simulink model "control_volume_two_phases_test01_sim"  (R2017b)
settings: Solver=ode23tb  StartTime=0.0  StopTime=400  MaxStep=0.2  RelTol=1e-3
undefined symbols (not defined in the file or in its folder): h, P, T
libraries: thermochemical x6, simulink x2
settings Model: Creator=ferru  LastModifiedBy=fferrucc
settings SolverCC: AlgebraicLoopSolver=LineSearch

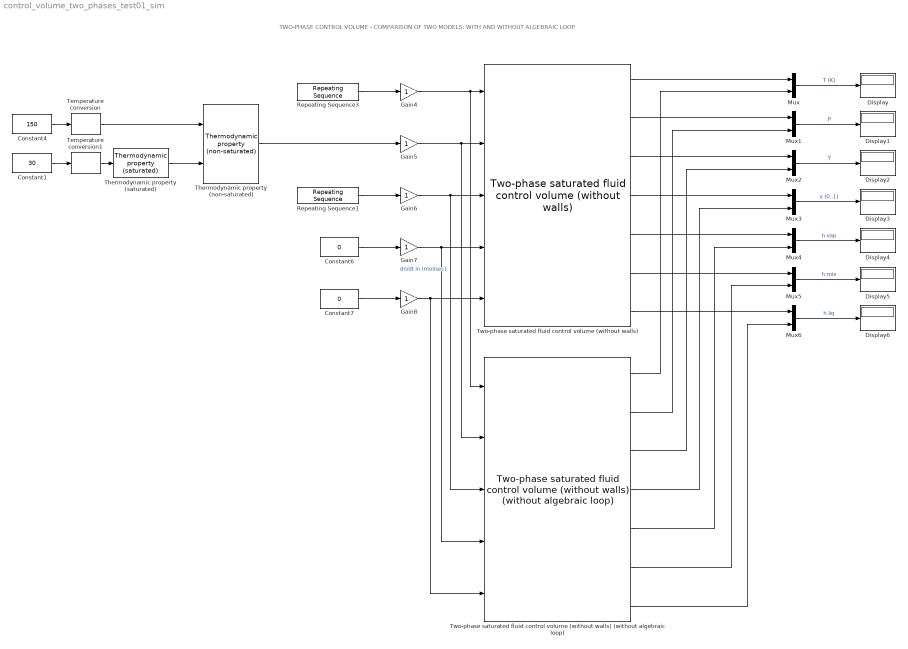
== system control_volume_two_phases_test01_sim ==
  note: TWO-PHASE CONTROL VOLUME - COMPARISON OF TWO MODELS: WITH AND WITHOUT ALGEBRAIC LOOP
  Constant1 : Constant  Value=30
  Constant4 : Constant  Value=150
  Constant6 : Constant  Value=0
  Constant7 : Constant  Value=0
  Display{,1..6} (7 alike) : Display
  Gain{4..8} (5 alike) : Gain
  Mux{,1..6} (7 alike) : Mux  Inputs=2
  Repeating Sequence1 : simulink/Sources/Repeating Sequence  rep_seq_t=[0, 100, 101, 200, 201]  rep_seq_y=[0, 0, 1, 1, 0]*0.02
  Repeating Sequence3 : simulink/Sources/Repeating Sequence  rep_seq_t=[0, 100, 101, 200, 201]  rep_seq_y=[1, 1, 0, 0, 1]*100
  Temperature conversion : thermochemical/Conversions/Temperature conversion  sel=°C --> K
      settings: SourceProductName=@ Thermochemical
  Temperature conversion1 : thermochemical/Conversions/Temperature conversion  sel=°C --> K
      settings: SourceProductName=@ Thermochemical
  Thermodynamic property (non-saturated) : thermochemical/Thermodynamic fluid properties/Thermodynamic  property (non-saturated)  sel=h(T,P)  fluid=nh3_v4  reciprocVar=-1  lookup2D_BreakPoint1=nh3_v4.no_sat.T_P_indep.var_indep.T  lookup2D_BreakPoint2=nh3_v4.no_sat.T_P_indep.var_indep.P  lookup2D_Data=nh3_v4.no_sat.T_P_indep.var_dep.h_molar
      settings: SourceProductName=@ Thermochemical
  Thermodynamic property (saturated) : thermochemical/Thermodynamic fluid properties/Thermodynamic  property (saturated)  sel=P(T) (bar)  fluid=nh3_v4  lookup1D_BreakPoint1=nh3_v4.sat.T  lookup1D_Data=nh3_v4.sat.Psat
      settings: SourceProductName=@ Thermochemical
  Two-phase saturated fluid control volume (without walls) : thermochemical/Control volumes/Two-phase saturated fluid control volume (without walls)  N_init=100  T_init=300  fluid=nh3_v4  V=0.01
      settings: SourceProductName=@ Thermochemical
  Two-phase saturated fluid control volume (without walls) (without algebraic loop) : thermochemical/Control volumes/Two-phase saturated fluid control volume (without walls) (without algebraic loop)  N_init=100  T_init=300  fluid=nh3_v4  V=0.01
      settings: SourceProductName=@ Thermochemical
  wires:
  Thermodynamic property (non-saturated)/1 -> Gain5/1
  Mux/1 -> Display/1  "T (K)"
  Two-phase saturated fluid control volume (without walls)/1 -> Mux/1
  Two-phase saturated fluid control volume (without walls) (without algebraic loop)/1 -> Mux/2
  Mux1/1 -> Display1/1  "P"
  Two-phase saturated fluid control volume (without walls)/2 -> Mux1/1
  Two-phase saturated fluid control volume (without walls) (without algebraic loop)/2 -> Mux1/2
  Mux3/1 -> Display3/1  "x (0..1)"
  Mux2/1 -> Display2/1  "Y"
  Two-phase saturated fluid control volume (without walls)/3 -> Mux2/1
  Two-phase saturated fluid control volume (without walls) (without algebraic loop)/3 -> Mux2/2
  Two-phase saturated fluid control volume (without walls)/4 -> Mux3/1
  Two-phase saturated fluid control volume (without walls) (without algebraic loop)/4 -> Mux3/2
  Mux5/1 -> Display5/1  "h mix"
  Mux6/1 -> Display6/1  "h liq"
  Mux4/1 -> Display4/1  "h vap"
  Two-phase saturated fluid control volume (without walls)/5 -> Mux4/1
  Two-phase saturated fluid control volume (without walls) (without algebraic loop)/5 -> Mux4/2
  Two-phase saturated fluid control volume (without walls)/6 -> Mux5/1
  Two-phase saturated fluid control volume (without walls) (without algebraic loop)/6 -> Mux5/2
  Two-phase saturated fluid control volume (without walls)/7 -> Mux6/1
  Two-phase saturated fluid control volume (without walls) (without algebraic loop)/7 -> Mux6/2
  Gain4/1 -> Two-phase saturated fluid control volume (without walls) (without algebraic loop)/1, Two-phase saturated fluid control volume (without walls)/1
  Gain5/1 -> Two-phase saturated fluid control volume (without walls) (without algebraic loop)/2, Two-phase saturated fluid control volume (without walls)/2
  Gain7/1 -> Two-phase saturated fluid control volume (without walls) (without algebraic loop)/4, Two-phase saturated fluid control volume (without walls)/4
  Gain6/1 -> Two-phase saturated fluid control volume (without walls) (without algebraic loop)/3, Two-phase saturated fluid control volume (without walls)/3  "dn/dt in (mol/sec)"
  Gain8/1 -> Two-phase saturated fluid control volume (without walls) (without algebraic loop)/5, Two-phase saturated fluid control volume (without walls)/5
  Constant6/1 -> Gain7/1
  Constant7/1 -> Gain8/1
  Thermodynamic property (saturated)/1 -> Thermodynamic property (non-saturated)/2
  Constant1/1 -> Temperature conversion1/1
  Constant4/1 -> Temperature conversion/1
  Temperature conversion/1 -> Thermodynamic property (non-saturated)/1
  Temperature conversion1/1 -> Thermodynamic property (saturated)/1
  Repeating Sequence1/1 -> Gain6/1
  Repeating Sequence3/1 -> Gain4/1
